simulink subsystem "PvtSubSys_VSM_LDW"  (R2020b)
settings: Solver=VariableStepAuto  StartTime=0.0  StopTime=10.0  RelTol=1e-3
values from neighbouring files (symbols this model uses):
  P_VSM_LDW_AbsEspInTime = 3.0    [LDW.sldd]
  P_VSM_LDW_absLongitudeAccIn = 2.5    [LDW.sldd]
  P_VSM_LDW_absLongitudeAccOut = 3.0    [LDW.sldd]
  P_VSM_LDW_AccPedalOut = 30.0    [LDW.sldd]
  P_VSM_LDW_AccRateIn = 30.0    [LDW.sldd]
  P_VSM_LDW_AccRateInTime = 1.5    [LDW.sldd]
  P_VSM_LDW_AccRateOut = 80.0    [LDW.sldd]
  P_VSM_LDW_AccRateOutTime = 0.0    [LDW.sldd]
  P_VSM_LDW_BrakePressIn = 3.0    [LDW.sldd]
  P_VSM_LDW_BrakePressInTime = 1.5    [LDW.sldd]
  P_VSM_LDW_BrakePressOut = 5.0    [LDW.sldd]
  P_VSM_LDW_LaneChangeOffset = 0.11    [LDW.sldd]
  P_VSM_LDW_LaneCurveIn = 0.005    [LDW.sldd]
  P_VSM_LDW_LaneCurveOut = 0.006    [LDW.sldd]
  P_VSM_LDW_LateralAcceIn = 3.0    [LDW.sldd]
  P_VSM_LDW_LateralAcceInTime = 3.0    [LDW.sldd]
  P_VSM_LDW_LateralAcceOut = 3.5    [LDW.sldd]
  P_VSM_LDW_LongitudeAccIn = 3.0    [LDW.sldd]
  P_VSM_LDW_LongitudeAccInTime = 3.0    [LDW.sldd]
  P_VSM_LDW_LongitudeAccOut = 3.5    [LDW.sldd]
  P_VSM_LDW_State_Absesp_enable = 1.0    [LDW.sldd]
  P_VSM_LDW_State_Accpedalrate_enable = 1.0    [LDW.sldd]
  P_VSM_LDW_State_Breakpressure_enable = 1.0    [LDW.sldd]
  P_VSM_LDW_State_ESSSts_enable = 1.0    [LDW.sldd]
  P_VSM_LDW_State_Failsafe_enable = 1.0    [LDW.sldd]
  P_VSM_LDW_State_GEAR_enable = 1.0    [LDW.sldd]
  P_VSM_LDW_State_Headingangle_enable = 1.0    [LDW.sldd]
  P_VSM_LDW_State_Lane_enable = 1.0    [LDW.sldd]
  P_VSM_LDW_State_LaneChange_enable = 1.0    [LDW.sldd]
  P_VSM_LDW_State_Lanecurve_enable = 1.0    [LDW.sldd]
  P_VSM_LDW_State_LateralAcce_enable = 1.0    [LDW.sldd]
  P_VSM_LDW_State_LongitudeAcc_enable = 1.0    [LDW.sldd]
  P_VSM_LDW_State_Param_LaneWidth_Offset : value not decoded    [LDW.sldd]
  P_VSM_LDW_State_Param_REWarningZoneIn = 0.35    [LDW.sldd]
  P_VSM_LDW_State_Param_Sensitive_Offset : value not decoded    [LDW.sldd]
  P_VSM_LDW_State_Param_WarningZoneIn = 0.2    [LDW.sldd]
  P_VSM_LDW_State_Param_WarningZoneOut = -0.65    [LDW.sldd]
  P_VSM_LDW_State_SteerWheelAngle_enable = 1.0    [LDW.sldd]
  P_VSM_LDW_State_SteerWheelSpd_enable = 1.0    [LDW.sldd]
  P_VSM_LDW_State_TurnLight_enable = 1.0    [LDW.sldd]
  P_VSM_LDW_State_Vehspeed_enable = 1.0    [LDW.sldd]
  P_VSM_LDW_State_Yawsup_enable = 1.0    [LDW.sldd]
  P_VSM_LDW_SteerWheelAngleIn = 70.0    [LDW.sldd]
  P_VSM_LDW_SteerWheelAngleInTime = 3.0    [LDW.sldd]
  P_VSM_LDW_SteerWheelAngleOut = 90.0    [LDW.sldd]
  P_VSM_LDW_SteerWheelSpdIn = 150.0    [LDW.sldd]
  P_VSM_LDW_SteerWheelSpdInTime = 3.0    [LDW.sldd]
  P_VSM_LDW_SteerWheelSpdOut = 200.0    [LDW.sldd]
  P_VSM_LDW_TurnLightInTime = 3.0    [LDW.sldd]
  P_VSM_LDW_WhelDy = 2.0    [LDW.sldd]
  P_VSM_LDW_YawRateIn = 0.2    [LDW.sldd]
  P_VSM_LDW_YawRateInTime = 1.0    [LDW.sldd]
  P_VSM_LDW_YawRateOut = 0.25    [LDW.sldd]
undefined symbols (not defined in the file or in its folder): P_VSM_LSMC_SampleTime
libraries: simulink x106
(part 2 of 3)

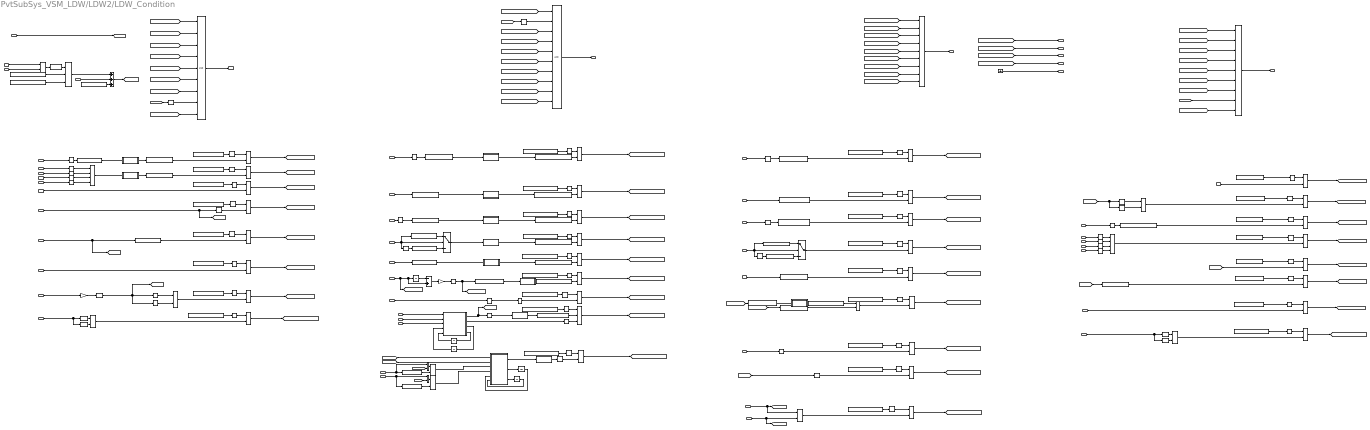
== system PvtSubSys_VSM_LDW/LDW2/LDW_Condition ==
  note: Ready2Active
  note: 0x0:Current gear "N" or "P"
      | 0x1:Current gear "1"
      | 0x2:Current gear "2"
      | 0x3:Current gear "3"
      | 0x4:Current gear "4"
      | 0x5:Current gear "5"
      | 0x6:Current gear "6"
      | 0x7:Current gear "7"
      | 0x8:Current gear "R"
      | 0x9-0xF:Reserved
  note: Active2Ready
  note: 0.2
  note: 0.35
  HWAActive : Inport
  canSASSteerWheelAngle : Inport  Port=2
  canSASSteerWheelSpd : Inport  Port=3
  canABMLateralAcce : Inport  Port=4
  LongitudeAcc : Inport  Port=5
  canESP_MasterCylindBrakePress : Inport  Port=6
  canECMAccrPedlPosnDiagc : Inport  Port=7
  CURRENT_GEAR : Inport  Port=8
  canBCMLeftTurnSWSts : Inport  Port=9
  canBCMRightTurnSWSts : Inport  Port=10
  Scene_LaneValid : Inport  Port=11
  canABMVehDynYawRate1 : Inport  Port=12
  canESPVDCActive1 : Inport  Port=13
  canESPPTCActive1 : Inport  Port=14
  canESPBTCActive1 : Inport  Port=15
  canABSABSActive1 : Inport  Port=16
  Common_Lane_Out : Inport  Port=17
  canABSVehicleSpd : Inport  Port=18
  Common_Lane_in : Inport  Port=19
  Headingangle_In : Inport  Port=20
  Headingangle_Out : Inport  Port=21
  LaneCurve : Inport  Port=22
  IFC_Failsafe : Inport  Port=23
  LeftChange : Inport  Port=24
  RightChange : Inport  Port=25
  FLWhelDy : Inport  Port=26
  FRWhelDy : Inport  Port=27
  ESSSts : Inport  Port=28
  LDWOffset : Inport  Port=29
  Host_LRE : Inport  Port=30
  Host_RRE : Inport  Port=31
  Abs{,1,3,6..8,11,15..16} (9 alike) : Abs
  Add : Sum  Inputs=-+
  Add1 : Sum  Inputs=+++
  Bias : Bias  Bias=1.3
  CURRENT_GEAR1 : InportShadow  Port=8
  Compare To Constant{1,19,24,28,32..33,38,42..44,46..48,56,69,78..79,82,88,115,118..119} (22 alike) : simulink/Logic and Bit Operations/Compare To Constant  relop===  const=1  OutDataTypeStr=boolean
  Compare To Constant{2,5..12,16..18,26..27,36,41,50..52,95,98,108,121,124} (24 alike) : simulink/Logic and Bit Operations/Compare To Constant  relop===  const=0  OutDataTypeStr=boolean
  Compare To Constant100 : simulink/Logic and Bit Operations/Compare To Constant  relop=<  const=P_VSM_LDW_LateralAcceIn  OutDataTypeStr=boolean
  Compare To Constant120 : simulink/Logic and Bit Operations/Compare To Constant  relop=>  const=P_VSM_LDW_AbsEspInTime  OutDataTypeStr=boolean
  Compare To Constant13 : simulink/Logic and Bit Operations/Compare To Constant  relop=>  const=0  OutDataTypeStr=boolean
  Compare To Constant14 : simulink/Logic and Bit Operations/Compare To Constant  relop=>  const=P_VSM_LDW_AccRateInTime  OutDataTypeStr=boolean
  Compare To Constant15 : simulink/Logic and Bit Operations/Compare To Constant  relop=>  const=P_VSM_LDW_TurnLightInTime  OutDataTypeStr=boolean
  Compare To Constant20 : simulink/Logic and Bit Operations/Compare To Constant  relop=<  const=P_VSM_LDW_BrakePressIn  OutDataTypeStr=boolean
  Compare To Constant21 : simulink/Logic and Bit Operations/Compare To Constant  relop===  const=8  OutDataTypeStr=boolean
  Compare To Constant22 : simulink/Logic and Bit Operations/Compare To Constant  relop=<  const=P_VSM_LDW_YawRateIn  OutDataTypeStr=boolean
  Compare To Constant23 : simulink/Logic and Bit Operations/Compare To Constant  relop=>  const=P_VSM_LDW_YawRateInTime  OutDataTypeStr=boolean
  Compare To Constant29 : simulink/Logic and Bit Operations/Compare To Constant  relop=<  const=P_VSM_LDW_SteerWheelAngleIn  OutDataTypeStr=boolean
  Compare To Constant3 : simulink/Logic and Bit Operations/Compare To Constant  relop=>  const=P_VSM_LDW_AccPedalOut  OutDataTypeStr=boolean
  Compare To Constant31 : simulink/Logic and Bit Operations/Compare To Constant  relop=<  const=P_VSM_LDW_SteerWheelSpdIn  OutDataTypeStr=boolean
  Compare To Constant35 : simulink/Logic and Bit Operations/Compare To Constant  relop=>  const=60  OutDataTypeStr=boolean
  Compare To Constant37 : simulink/Logic and Bit Operations/Compare To Constant  relop=<  const=150  OutDataTypeStr=boolean
  Compare To Constant39 : simulink/Logic and Bit Operations/Compare To Constant  relop=<  const=55  OutDataTypeStr=boolean
  Compare To Constant4 : simulink/Logic and Bit Operations/Compare To Constant  relop=>  const=P_VSM_LDW_AccRateOutTime  OutDataTypeStr=boolean
  Compare To Constant40 : simulink/Logic and Bit Operations/Compare To Constant  relop=>  const=155  OutDataTypeStr=boolean
  Compare To Constant49 : simulink/Logic and Bit Operations/Compare To Constant  relop=>  const=0.5  OutDataTypeStr=boolean
  Compare To Constant53 : simulink/Logic and Bit Operations/Compare To Constant  relop=~=  const=5  OutDataTypeStr=boolean
  Compare To Constant54 : simulink/Logic and Bit Operations/Compare To Constant  relop=<  const=P_VSM_LDW_WhelDy  OutDataTypeStr=boolean
  Compare To Constant55 : simulink/Logic and Bit Operations/Compare To Constant  relop=<  const=P_VSM_LDW_WhelDy  OutDataTypeStr=boolean
  Compare To Constant57 : simulink/Logic and Bit Operations/Compare To Constant  relop===  const=8  OutDataTypeStr=boolean
  Compare To Constant58 : simulink/Logic and Bit Operations/Compare To Constant  relop=<  const=P_VSM_LDW_LongitudeAccIn  OutDataTypeStr=boolean
  Compare To Constant59 : simulink/Logic and Bit Operations/Compare To Constant  relop=<  const=P_VSM_LDW_absLongitudeAccIn  OutDataTypeStr=boolean
  Compare To Constant60 : simulink/Logic and Bit Operations/Compare To Constant  relop===  const=5  OutDataTypeStr=boolean
  Compare To Constant61 : simulink/Logic and Bit Operations/Compare To Constant  relop=>  const=P_VSM_LDW_SteerWheelAngleOut  OutDataTypeStr=boolean
  Compare To Constant62 : simulink/Logic and Bit Operations/Compare To Constant  relop===  const=4  OutDataTypeStr=boolean
  Compare To Constant63 : simulink/Logic and Bit Operations/Compare To Constant  relop=<  const=P_VSM_LDW_LaneCurveIn  OutDataTypeStr=boolean
  Compare To Constant65 : simulink/Logic and Bit Operations/Compare To Constant  relop=>  const=P_VSM_LDW_SteerWheelAngleInTime  OutDataTypeStr=boolean
  Compare To Constant67 : simulink/Logic and Bit Operations/Compare To Constant  relop=~=  const=4  OutDataTypeStr=boolean
  Compare To Constant70 : simulink/Logic and Bit Operations/Compare To Constant  relop=>  const=P_VSM_LDW_YawRateOut  OutDataTypeStr=boolean
  Compare To Constant73 : simulink/Logic and Bit Operations/Compare To Constant  relop=>  const=P_VSM_LDW_SteerWheelSpdOut  OutDataTypeStr=boolean
  Compare To Constant74 : simulink/Logic and Bit Operations/Compare To Constant  relop=>  const=P_VSM_LDW_SteerWheelSpdInTime  OutDataTypeStr=boolean
  Compare To Constant75 : simulink/Logic and Bit Operations/Compare To Constant  relop=>  const=P_VSM_LDW_LateralAcceOut  OutDataTypeStr=boolean
  Compare To Constant76 : simulink/Logic and Bit Operations/Compare To Constant  relop=>  const=P_VSM_LDW_LongitudeAccOut  OutDataTypeStr=boolean
  Compare To Constant77 : simulink/Logic and Bit Operations/Compare To Constant  relop=>  const=P_VSM_LDW_absLongitudeAccOut  OutDataTypeStr=boolean
  Compare To Constant80 : simulink/Logic and Bit Operations/Compare To Constant  relop=>  const=P_VSM_LDW_BrakePressOut  OutDataTypeStr=boolean
  Compare To Constant83 : simulink/Logic and Bit Operations/Compare To Constant  relop=>  const=P_VSM_LDW_AccRateOut  OutDataTypeStr=boolean
  Compare To Constant85 : simulink/Logic and Bit Operations/Compare To Constant  relop=>  const=P_VSM_LDW_LaneCurveOut  OutDataTypeStr=boolean
  Compare To Constant91 : simulink/Logic and Bit Operations/Compare To Constant  relop=<  const=P_VSM_LDW_AccRateIn  OutDataTypeStr=boolean
  Compare To Constant92 : simulink/Logic and Bit Operations/Compare To Constant  relop=>  const=P_VSM_LDW_BrakePressInTime  OutDataTypeStr=boolean
  Compare To Constant94 : simulink/Logic and Bit Operations/Compare To Constant  relop=>  const=P_VSM_LDW_LongitudeAccInTime  OutDataTypeStr=boolean
  Compare To Constant96 : simulink/Logic and Bit Operations/Compare To Constant  relop=>  const=P_VSM_LDW_LateralAcceInTime  OutDataTypeStr=boolean
  Constant : Constant  Value=P_VSM_LDW_LaneChangeOffset
  Data Type Conversion : DataTypeConversion
  ESSSts2 : InportShadow  Port=28
  Gain : Gain  Gain=1.03
  Gain1 : Gain  Gain=50
  Ground : Ground
  Logical Operator{,3,5,7,9..12,15,17,19..20,24..26,38..41,46,60,62} (22 alike) : Logic  AllPortsSameDT=off  OutDataTypeStr=boolean
  Logical Operator1 : Logic  Inputs=4  AllPortsSameDT=off  OutDataTypeStr=boolean
  Logical Operator13 : Logic  Operator=OR  Inputs=4  AllPortsSameDT=off  OutDataTypeStr=boolean
  Logical Operator{4,6,8,16,18,21..22,27,29..32,34,36..37,42,49,52,59,61} (20 alike) : Logic  Operator=OR  AllPortsSameDT=off  OutDataTypeStr=boolean
  Logical Operator23 : Logic  Operator=NOT  AllPortsSameDT=off  OutDataTypeStr=boolean
  Logical Operator35 : Logic  Operator=NOT  AllPortsSameDT=off  OutDataTypeStr=boolean
  Logical Operator43 : Logic  Operator=OR  Inputs=9  AllPortsSameDT=off  OutDataTypeStr=boolean
  Logical Operator45 : Logic  Operator=OR  Inputs=9  AllPortsSameDT=off  OutDataTypeStr=boolean
  Logical Operator51 : Logic  Operator=OR  Inputs=3  AllPortsSameDT=off  OutDataTypeStr=boolean
  Logical Operator86 : Logic  Inputs=9  AllPortsSameDT=off  OutDataTypeStr=boolean
  Logical Operator94 : Logic  Inputs=10  AllPortsSameDT=off  OutDataTypeStr=boolean
  LongitudeAcc1 : InportShadow  Port=5
  MATLAB Function : MATLAB Function  TreatAsAtomicUnit=on
  Multiport Switch : MultiPortSwitch  Inputs=2  DiagnosticForDefault=None
  Relational Operator : RelationalOperator  OutDataTypeStr=boolean  RndMeth=Simplest
  Relational Operator1 : RelationalOperator  OutDataTypeStr=boolean  RndMeth=Simplest
  State_TurnLight2 : MATLAB Function  TreatAsAtomicUnit=on
  Subsystem : Subsystem  mask{Ts=P_VSM_LSMC_SampleTime, Max=10}
      mask prompts: Ts "Sample Time:"; Max "Max Limit:"
      mask Display:
      | Ts=get_param(gcb,'Ts');
      | Max=get_param(gcb,'Max');
      | disp(['Ts:' Ts '\n' 'Max:' Max ]);
  Subsystem1 : Subsystem  mask{Ts=P_VSM_LSMC_SampleTime, Max=10}
      mask prompts: Ts "Sample Time:"; Max "Max Limit:"
      mask Display:
      | Ts=get_param(gcb,'Ts');
      | Max=get_param(gcb,'Max');
      | disp(['Ts:' Ts '\n' 'Max:' Max ]);
  Subsystem10 : Subsystem  mask{Ts=P_VSM_LSMC_SampleTime, Max=10}
      mask prompts: Ts "Sample Time:"; Max "Max Limit:"
      mask Display:
      | Ts=get_param(gcb,'Ts');
      | Max=get_param(gcb,'Max');
      | disp(['Ts:' Ts '\n' 'Max:' Max ]);
  Subsystem17 : Subsystem  mask{Ts=P_VSM_LSMC_SampleTime, Max=10}
      mask prompts: Ts "Sample Time:"; Max "Max Limit:"
      mask Display:
      | Ts=get_param(gcb,'Ts');
      | Max=get_param(gcb,'Max');
      | disp(['Ts:' Ts '\n' 'Max:' Max ]);
  Subsystem2 : Subsystem  mask{Ts=P_VSM_LSMC_SampleTime, Max=10}
      mask prompts: Ts "Sample Time:"; Max "Max Limit:"
      mask Display:
      | Ts=get_param(gcb,'Ts');
      | Max=get_param(gcb,'Max');
      | disp(['Ts:' Ts '\n' 'Max:' Max ]);
  Subsystem3 : Subsystem  mask{Ts=P_VSM_LSMC_SampleTime, Max=10}
      mask prompts: Ts "Sample Time:"; Max "Max Limit:"
      mask Display:
      | Ts=get_param(gcb,'Ts');
      | Max=get_param(gcb,'Max');
      | disp(['Ts:' Ts '\n' 'Max:' Max ]);
  Subsystem4 : Subsystem  mask{Ts=P_VSM_LSMC_SampleTime, Max=10}
      mask prompts: Ts "Sample Time:"; Max "Max Limit:"
      mask Display:
      | Ts=get_param(gcb,'Ts');
      | Max=get_param(gcb,'Max');
      | disp(['Ts:' Ts '\n' 'Max:' Max ]);
  Subsystem5 : Subsystem  mask{Ts=P_VSM_LSMC_SampleTime, Max=10}
      mask prompts: Ts "Sample Time:"; Max "Max Limit:"
      mask Display:
      | Ts=get_param(gcb,'Ts');
      | Max=get_param(gcb,'Max');
      | disp(['Ts:' Ts '\n' 'Max:' Max ]);
  Subsystem6 : Subsystem  mask{Ts=P_VSM_LSMC_SampleTime, Max=10}
      mask prompts: Ts "Sample Time:"; Max "Max Limit:"
      mask Display:
      | Ts=get_param(gcb,'Ts');
      | Max=get_param(gcb,'Max');
      | disp(['Ts:' Ts '\n' 'Max:' Max ]);
  Subsystem7 : Subsystem  mask{Ts=P_VSM_LSMC_SampleTime, Max=10}
      mask prompts: Ts "Sample Time:"; Max "Max Limit:"
      mask Display:
      | Ts=get_param(gcb,'Ts');
      | Max=get_param(gcb,'Max');
      | disp(['Ts:' Ts '\n' 'Max:' Max ]);
  Subsystem8 : Subsystem  mask{Ts=P_VSM_LSMC_SampleTime, Max=10}
      mask prompts: Ts "Sample Time:"; Max "Max Limit:"
      mask Display:
      | Ts=get_param(gcb,'Ts');
      | Max=get_param(gcb,'Max');
      | disp(['Ts:' Ts '\n' 'Max:' Max ]);
  Switch2 : Switch  Criteria=u2 > Threshold
  Switch4 : Switch  Criteria=u2 > Threshold
  Unit Delay{1..4,8} (5 alike) : UnitDelay  SampleTime=-1  HasFrameUpgradeWarning=on
  WarningZoneIn : Constant  Value=P_VSM_LDW_State_Param_WarningZoneIn
  WarningZoneIn1 : Constant  Value=P_VSM_LDW_State_Param_REWarningZoneIn
  canABMLateralAcce2 : InportShadow  Port=4
  canABMVehDynYawRate2 : InportShadow  Port=12
  canABSABSActive2 : InportShadow  Port=16
  canESPBTCActive2 : InportShadow  Port=15
  canESPPTCActive2 : InportShadow  Port=14
  canESPVDCActive2 : InportShadow  Port=13
  canESP_MasterCylindBrakePress2 : InportShadow  Port=6
  canSASSteerWheelAngle1 : InportShadow  Port=2
  canSASSteerWheelSpd2 : InportShadow  Port=3
  param_1 : Constant  Value=P_VSM_LDW_State_SteerWheelAngle_enable
  param_10 : Constant  Value=P_VSM_LDW_State_Headingangle_enable
  param_11 : Constant  Value=P_VSM_LDW_State_Breakpressure_enable
  param_13 : Constant  Value=P_VSM_LDW_State_Accpedalrate_enable
  param_14 : Constant  Value=P_VSM_LDW_State_Absesp_enable
  param_15 : Constant  Value=P_VSM_LDW_State_Failsafe_enable
  param_17 : Constant  Value=P_VSM_LDW_State_Lanecurve_enable
  param_18 : Constant  Value=P_VSM_LDW_State_GEAR_enable
  param_19 : Constant  Value=P_VSM_LDW_State_ESSSts_enable
  param_2 : Constant  Value=P_VSM_LDW_State_LaneChange_enable
  param_20 : Constant  Value=P_VSM_LDW_State_TurnLight_enable
  param_23 : Constant  Value=P_VSM_LDW_State_SteerWheelSpd_enable
  param_24 : Constant  Value=P_VSM_LDW_State_LateralAcce_enable
  param_25 : Constant  Value=P_VSM_LDW_State_Vehspeed_enable
  param_26 : Constant  Value=P_VSM_LDW_State_Yawsup_enable
  param_27 : Constant  Value=P_VSM_LDW_State_Absesp_enable
  param_28 : Constant  Value=P_VSM_LDW_State_LongitudeAcc_enable
  param_29 : Constant  Value=P_VSM_LDW_State_Lane_enable
  param_3 : Constant  Value=P_VSM_LDW_State_Yawsup_enable
  param_30 : Constant  Value=P_VSM_LDW_State_Failsafe_enable
  param_31 : Constant  Value=P_VSM_LDW_State_Breakpressure_enable
  param_32 : Constant  Value=P_VSM_LDW_State_Headingangle_enable
  param_33 : Constant  Value=P_VSM_LDW_State_Lanecurve_enable
  param_4 : Constant  Value=P_VSM_LDW_State_SteerWheelAngle_enable
  param_40 : Constant  Value=P_VSM_LDW_State_Lane_enable
  param_42 : Constant  Value=P_VSM_LDW_State_Vehspeed_enable
  param_43 : Constant  Value=P_VSM_LDW_State_Accpedalrate_enable
  param_45 : Constant  Value=P_VSM_LDW_State_GEAR_enable
  param_46 : Constant  Value=P_VSM_LDW_State_TurnLight_enable
  param_47 : Constant  Value=P_VSM_LDW_State_LaneChange_enable
  param_6 : Constant  Value=P_VSM_LDW_State_SteerWheelSpd_enable
  param_7 : Constant  Value=P_VSM_LDW_State_LateralAcce_enable
  param_8 : Constant  Value=P_VSM_LDW_State_ESSSts_enable
  param_9 : Constant  Value=P_VSM_LDW_State_LongitudeAcc_enable
  LDW_Idle2Ready : Outport
  LDW_Ready2Active : Outport  Port=2
  LDW_Active2Ready : Outport  Port=3
  LDW_Ready2Idle_Active2Idle : Outport  Port=4
  LDW_Con_AccPedalRate_LDWExit : Outport  Port=5
  LDW_Con_BrakePressure_ LDWExit : Outport  Port=6
  LDW_Con_SteerWheelSpd_ LDWExit : Outport  Port=7
  LDW_Con_SteerWheelAngle_ LDWExit : Outport  Port=8
  LDW_Con_DriverInput_ LDWExit : Outport  Port=9
  wires:
  LDWOffset/1 -> Add1/2
  [Con_AccPedalRate_Active2Ready] -> LDW_Con_AccPedalRate_LDWExit/1  "LDW_Con_AccPedalRate_LDWExit"
  Ground/1 -> LDW_Con_DriverInput_ LDWExit/1  "LDW_Con_DriverInput_ LDWExit"
  [Con_SteerWheelAngle_Active2Ready] -> LDW_Con_SteerWheelAngle_ LDWExit/1  "LDW_Con_SteerWheelAngle_ LDWExit"
  [Con_SteerWheelSpd_Active2Ready] -> LDW_Con_SteerWheelSpd_ LDWExit/1  "LDW_Con_SteerWheelSpd_ LDWExit"
  [Con_BrakePressure_Active2Ready] -> LDW_Con_BrakePressure_ LDWExit/1  "LDW_Con_BrakePressure_ LDWExit"
  [Con_SteerWheelSpd_Ready2Active] -> Logical Operator94/3
  [Con_BrakePressure_Ready2Active] -> Logical Operator94/6
  [Con_LateralAcc_Ready2Active] -> Logical Operator94/4
  [Con_AccPedalRate_Ready2Active] -> Logical Operator94/7
  [Con_SteerWheelAngle_Ready2Active] -> Logical Operator94/1
  canBCMLeftTurnSWSts/1 -> State_TurnLight2/1(leftlight)
  Compare To Constant42/1 -> Logical Operator10/1
  Compare To Constant2/1 -> Logical Operator27/1
  Compare To Constant13/1 -> Logical Operator15/2
  Compare To Constant47/1 -> Logical Operator15/1
  Logical Operator27/1 -> [Con_SteerWheelAngle_Ready2Active]  "VSM_LDW_Con_SteerWheelAngle_Ready2Active"
  Logical Operator17/1 -> [Con_CURRENT_GEAR_Active2Ready]  "VSM_LDW_Con_CURRENT_GEAR_Active2Ready"
  Compare To Constant27/1 -> Logical Operator51/1
  LongitudeAcc/1 -> Switch2/2, Compare To Constant58/1, Abs7/1
  Compare To Constant59/1 -> Switch2/3
  Logical Operator3/1 -> [Con_SteerWheelSpd_Active2Ready]  "VSM_LDW_Con_SteerWheelSpd_Active2Ready"
  Compare To Constant8/1 -> Logical Operator31/1
  canSASSteerWheelAngle1/1 -> Abs8/1
  Abs16/1 -> Compare To Constant75/1
  CURRENT_GEAR1/1 -> Compare To Constant57/1
  Logical Operator11/1 -> [Con_BrakePressure_Active2Ready]  "VSM_LDW_Con_BrakePressure_Active2Ready"
  param_20/1 -> Compare To Constant27/1
  Switch4/1 -> Logical Operator10/2
  Logical Operator35/1 -> Logical Operator37/2
  Compare To Constant77/1 -> Switch4/3
  LongitudeAcc1/1 -> Abs15/1, Compare To Constant76/1, Switch4/2
  Abs3/1 -> [AccrPedlPosnRate], Compare To Constant91/1
  Compare To Constant124/1 -> Logical Operator52/1
  Logical Operator31/1 -> [Con_SteerWheelSpd_Ready2Active]  "VSM_LDW_Con_SteerWheelSpd_Ready2Active"
  Abs7/1 -> Compare To Constant59/1
  Abs8/1 -> Compare To Constant61/1
  canESP_MasterCylindBrakePress2/1 -> Compare To Constant80/1
  [AccrPedlPosnRate] -> Compare To Constant83/1
  Compare To Constant33/1 -> Logical Operator12/1
  Compare To Constant78/1 -> Logical Operator11/1
  CURRENT_GEAR/1 -> Compare To Constant21/1
  Compare To Constant75/1 -> Logical Operator7/2
  Logical Operator10/1 -> [Con_LongitudeAcc_Active2Ready]  "VSM_LDW_Con_LongitudeAcc_Active2Ready"
  Compare To Constant46/1 -> Logical Operator38/1
  Logical Operator37/1 -> [Con_CURRENT_GEAR_Ready2Active]  "VSM_LDW_Con_CURRENT_GEAR_Ready2Active"
  Abs1/1 -> Compare To Constant29/1
  Compare To Constant58/1 -> Switch2/1
  param_1/1 -> Compare To Constant2/1
  Logical Operator7/1 -> [Con_LateralAcc_Active2Ready]  "VSM_LDW_Con_LateralAcc_Active2Ready"
  Compare To Constant61/1 -> Logical Operator38/2
  Compare To Constant21/1 -> Logical Operator35/1
  canBCMRightTurnSWSts/1 -> State_TurnLight2/2(rightlight)
  canESP_MasterCylindBrakePress/1 -> Compare To Constant20/1
  canABMLateralAcce2/1 -> Abs16/1
  Abs11/1 -> Compare To Constant100/1
  Logical Operator49/1 -> [Con_BrakePressure_Ready2Active]  "VSM_LDW_Con_BrakePressure_Ready2Active"
  Compare To Constant121/1 -> Logical Operator49/1
  Abs15/1 -> Compare To Constant77/1
  canSASSteerWheelSpd2/1 -> Compare To Constant73/1
  canABMLateralAcce/1 -> Abs11/1
  Compare To Constant11/1 -> Logical Operator34/1
  Logical Operator52/1 -> [Con_AccPedalRate_Ready2Active]  "VSM_LDW_Con_AccPedalRate_Ready2Active"
  param_6/1 -> Compare To Constant8/1
  Logical Operator38/1 -> [Con_SteerWheelAngle_Active2Ready]  "VSM_LDW_Con_SteerWheelAngle_Active2Ready"
  [Con_LongitudeAcc_Ready2Active] -> Logical Operator94/5
  Compare To Constant73/1 -> Logical Operator3/2
  Logical Operator32/1 -> [Con_LateralAcc_Ready2Active]  "VSM_LDW_Con_LateralAcc_Ready2Active"
  Compare To Constant48/1 -> Logical Operator17/1
  Logical Operator34/1 -> [Con_LongitudeAcc_Ready2Active]  "VSM_LDW_Con_LongitudeAcc_Ready2Active"
  Logical Operator51/1 -> [Con_TurnLight_Ready2Active]  "VSM_LDW_Con_TurnLight_Ready2Active"
  Compare To Constant43/1 -> Logical Operator7/1
  canSASSteerWheelSpd/1 -> Compare To Constant31/1
  Compare To Constant26/1 -> Logical Operator37/1
  Compare To Constant9/1 -> Logical Operator32/1
  [Turnlight] -> Compare To Constant13/1
  Logical Operator15/1 -> [Con_TurnLight_Active2Ready]  "VSM_LDW_Con_TurnLight_Active2Ready"
  [Con_LateralAcc_Active2Ready] -> Logical Operator45/4
  Compare To Constant76/1 -> Switch4/1
  [Con_LaneChange_Active2Ready] -> Logical Operator45/8
  [Con_AccPedalRate_Active2Ready] -> Logical Operator45/7
  Logical Operator12/1 -> [Con_AccPedalRate_Active2Ready]  "VSM_LDW_Con_AccPedalRate_Active2Ready"
  [Con_BrakePressure_Active2Ready] -> Logical Operator45/6
  [Con_CURRENT_GEAR_Active2Ready] -> Logical Operator45/2
  [Con_SteerWheelSpd_Active2Ready] -> Logical Operator45/3
  canSASSteerWheelAngle/1 -> Abs1/1
  [Con_SteerWheelAngle_Active2Ready] -> Logical Operator45/1
  Compare To Constant44/1 -> Logical Operator3/1
  [Con_LongitudeAcc_Active2Ready] -> Logical Operator45/5
  Compare To Constant57/1 -> Logical Operator17/2
  param_4/1 -> Compare To Constant46/1
  param_17/1 -> Compare To Constant115/1
  Logical Operator46/1 -> [Con_LaneCurve_Ready2Idle]  "VSM_LDW_Con_LaneCurve_Ready2Idle"
  Compare To Constant85/1 -> Logical Operator46/2
  Headingangle_Out/1 -> Logical Operator26/2
  Logical Operator26/1 -> [Con_Headingangle_Ready2Idle]  "VSM_LDW_Con_Headingangle_Ready2Idle"
  param_32/1 -> Compare To Constant32/1
  Compare To Constant40/1 -> Logical Operator61/2
  param_25/1 -> Compare To Constant38/1
  canABSABSActive1/1 -> Compare To Constant69/1
  canESPVDCActive1/1 -> Compare To Constant79/1
  Compare To Constant19/1 -> Logical Operator9/1
  Logical Operator39/1 -> [Con_YawRate_Ready2Idle]  "VSM_LDW_Con_YawRate_Ready2Idle"
  Logical Operator24/1 -> [Con_Failsafe_Ready2Idle]  "VSM_LDW_Con_Failsafe_Ready2Idle"
  Logical Operator40/1 -> [Con_AbsEsp_Ready2Idle]  "VSM_LDW_Con_AbsEsp_Ready2Idle"
  Compare To Constant39/1 -> Logical Operator61/1
  param_29/1 -> Compare To Constant19/1
  Compare To Constant115/1 -> Logical Operator46/1
  Compare To Constant88/1 -> Logical Operator13/3
  Compare To Constant70/1 -> Logical Operator39/2
  [IFC_Failsafe] -> Logical Operator24/2
  canABMVehDynYawRate1/1 -> Abs6/1
  Abs6/1 -> Compare To Constant70/1
  Logical Operator62/1 -> [Con_VehicleSpeed_Ready2Idle]  "VSM_LDW_Con_VehicleSpeed_Ready2Idle"
  Compare To Constant32/1 -> Logical Operator26/1
  Compare To Constant69/1 -> Logical Operator13/4
  param_30/1 -> Compare To Constant28/1
  canESPBTCActive1/1 -> Compare To Constant88/1
  Compare To Constant119/1 -> Logical Operator40/1
  param_27/1 -> Compare To Constant119/1
  Logical Operator13/1 -> Logical Operator40/2  "absespsup"
  Compare To Constant38/1 -> Logical Operator62/1
  Compare To Constant118/1 -> Logical Operator39/1
  Common_Lane_Out/1 -> Logical Operator9/2
  Logical Operator9/1 -> [Con_Lane_Ready2Idle]  "VSM_LDW_Con_Lane_Ready2Idle"
  param_26/1 -> Compare To Constant118/1
  Compare To Constant79/1 -> Logical Operator13/1
  Logical Operator61/1 -> Logical Operator62/2
  [LaneCurve] -> Compare To Constant85/1
  [Con_AbsEsp_Ready2Idle] -> Logical Operator43/2
  [speed] -> Compare To Constant39/1, Compare To Constant40/1
  [Con_Failsafe_Ready2Idle] -> Logical Operator43/3
  Compare To Constant82/1 -> Logical Operator13/2
  Compare To Constant28/1 -> Logical Operator24/1
  [Con_Headingangle_Ready2Idle] -> Logical Operator43/5
  [Con_YawRate_Ready2Idle] -> Logical Operator43/1
  canESPPTCActive1/1 -> Compare To Constant82/1
  Logical Operator43/1 -> LDW_Ready2Idle_Active2Idle/1  "VSM_LDW_Other2Idle"
  [Con_LaneCurve_Ready2Idle] -> Logical Operator43/4
  canABSVehicleSpd/1 -> Gain/1
  Logical Operator23/1 -> Logical Operator8/2
  [Con_Headingangel_Idle2Ready] -> Logical Operator86/3
  Common_Lane_in/1 -> Logical Operator4/2
  [Con_Failsafe_Idle2Ready] -> Logical Operator86/4
  Logical Operator86/1 -> LDW_Idle2Ready/1  "VSM_LDW_Idle2Ready"
  Compare To Constant35/1 -> Logical Operator60/1
  [Con_AbsEsp_Idle2Ready] -> Logical Operator86/2
  [Con_YawRate_Idle2Ready] -> Logical Operator86/1
  param_40/1 -> Compare To Constant16/1
  Logical Operator6/1 -> [Con_Headingangel_Idle2Ready]  "VSM_LDW_Con_Headingangle_Idle2Ready"
  Compare To Constant18/1 -> Logical Operator8/1
  param_15/1 -> Compare To Constant18/1
  Subsystem17/1(Out1) -> Compare To Constant120/1
  canABMVehDynYawRate2/1 -> Abs/1
  canESPBTCActive2/1 -> Compare To Constant7/1
  Subsystem/1(Out1) -> Compare To Constant23/1
  Compare To Constant22/1 -> Subsystem/1(In1)
  IFC_Failsafe/1 -> [IFC_Failsafe], Logical Operator23/1
  Logical Operator59/1 -> [Con_VehicleSpeed_Idle2Ready]  "VSM_LDW_Con_VehicleSpeed_Idle2Ready"
  param_33/1 -> Compare To Constant108/1
  Logical Operator29/1 -> [Con_YawRate_Idle2Ready]  "VSM_LDW_Con_YawRate_Idle2Ready"
  Logical Operator8/1 -> [Con_Failsafe_Idle2Ready]  "VSM_LDW_Con_Failsafe_Idle2Ready"
  Compare To Constant16/1 -> Logical Operator4/1
  Compare To Constant17/1 -> Logical Operator6/1
  canABSABSActive2/1 -> Compare To Constant10/1
  Compare To Constant5/1 -> Logical Operator1/1
  param_10/1 -> Compare To Constant17/1
  Compare To Constant6/1 -> Logical Operator1/2
  Compare To Constant7/1 -> Logical Operator1/3
  canESPVDCActive2/1 -> Compare To Constant5/1
  param_42/1 -> Compare To Constant36/1
  Logical Operator1/1 -> Subsystem17/1(In1)
  Compare To Constant95/1 -> Logical Operator29/1
  Bias/1 -> Compare To Constant35/1, Compare To Constant37/1, [speed]
  Compare To Constant37/1 -> Logical Operator60/2
  Compare To Constant36/1 -> Logical Operator59/1
  canESPPTCActive2/1 -> Compare To Constant6/1
  Logical Operator4/1 -> [Con_Lane_Idle2Ready]  "VSM_LDW_Con_Lane_Idle2Ready"
  Abs/1 -> Compare To Constant22/1
  param_3/1 -> Compare To Constant95/1
  Logical Operator36/1 -> [Con_LaneCurve_Idle2Ready]  "VSM_LDW_Con_LaneCurve_Idle2Ready"
  Compare To Constant108/1 -> Logical Operator36/1
  Compare To Constant98/1 -> Logical Operator30/1
  Logical Operator30/1 -> [Con_AbsEsp_Idle2Ready]  "VSM_LDW_Con_AbsEsp_Idle2Ready"
  LaneCurve/1 -> Compare To Constant63/1, [LaneCurve]
  Compare To Constant23/1 -> Logical Operator29/2
  Compare To Constant120/1 -> Logical Operator30/2
  Logical Operator60/1 -> Logical Operator59/2  "LogicalOperator60"
  Gain/1 -> Bias/1
  param_14/1 -> Compare To Constant98/1
  Compare To Constant63/1 -> Logical Operator36/2
  Compare To Constant10/1 -> Logical Operator1/4
  Logical Operator45/1 -> LDW_Active2Ready/1  "VSM_LDW_Active2Ready"
  Logical Operator94/1 -> LDW_Ready2Active/1  "VSM_LDW_Ready2Active"
  [Con_VehicleSpeed_Ready2Idle] -> Logical Operator43/6
  [Con_Lane_Ready2Idle] -> Logical Operator43/7
  Headingangle_In/1 -> Logical Operator6/2
  Compare To Constant15/1 -> Logical Operator51/2
  Compare To Constant12/1 -> Subsystem1/1(In1)
  Subsystem1/1(Out1) -> Compare To Constant15/1
  Compare To Constant14/1 -> Logical Operator52/2
  Compare To Constant80/1 -> Logical Operator11/2
  Compare To Constant92/1 -> Logical Operator49/2
  Compare To Constant94/1 -> Logical Operator34/2
  Compare To Constant91/1 -> Subsystem3/1(In1)
  Subsystem3/1(Out1) -> Compare To Constant14/1
  Compare To Constant20/1 -> Subsystem4/1(In1)
  Subsystem4/1(Out1) -> Compare To Constant92/1
  Switch2/1 -> Subsystem6/1(In1)
  Subsystem6/1(Out1) -> Compare To Constant94/1
  Compare To Constant96/1 -> Logical Operator32/2
  Compare To Constant100/1 -> Subsystem7/1(In1)
  Subsystem7/1(Out1) -> Compare To Constant96/1
  Compare To Constant74/1 -> Logical Operator31/2
  Subsystem10/1(Out1) -> Compare To Constant74/1
  Compare To Constant31/1 -> Subsystem10/1(In1)
  Compare To Constant65/1 -> Logical Operator27/2
  Compare To Constant29/1 -> Subsystem8/1(In1)
  Subsystem8/1(Out1) -> Compare To Constant65/1
  Compare To Constant24/1 -> Logical Operator5/1
  Logical Operator5/1 -> [Con_LaneChange_Active2Ready]  "VSM_LDW_Con_LaneChange_Active2Ready"
  Compare To Constant41/1 -> Logical Operator18/1
  Logical Operator18/1 -> [Con_LaneChange_Ready2Active]  "VSM_LDW_Con_LaneChange_Ready2Active"
  [Con_LaneCurve_Idle2Ready] -> Logical Operator86/5
  [Con_Lane_Idle2Ready] -> Logical Operator86/6
  [Con_VehicleSpeed_Idle2Ready] -> Logical Operator86/7
  Add/1 -> Gain1/1
  Gain1/1 -> Abs3/1
  Unit Delay4/1 -> Add/1
  [Con_CURRENT_GEAR_Ready2Active] -> Logical Operator94/8
  [Con_TurnLight_Ready2Active] -> Logical Operator94/9
  Compare To Constant1/1 -> Logical Operator51/3
  [Con_LaneChange_Ready2Active] -> Logical Operator94/10
  State_TurnLight2/3(left) -> Unit Delay8/1
  Unit Delay8/1 -> State_TurnLight2/4(leftk1)
  State_TurnLight2/4(right) -> Unit Delay1/1
  Unit Delay1/1 -> State_TurnLight2/5(rightk1)
  Scene_LaneValid/1 -> State_TurnLight2/3(lane)
  param_7/1 -> Compare To Constant9/1
  param_9/1 -> Compare To Constant11/1
  param_11/1 -> Compare To Constant121/1
  param_13/1 -> Compare To Constant124/1
  param_18/1 -> Compare To Constant26/1
  param_2/1 -> Compare To Constant41/1
  param_23/1 -> Compare To Constant44/1
  param_24/1 -> Compare To Constant43/1
  param_28/1 -> Compare To Constant42/1
  param_31/1 -> Compare To Constant78/1
  param_43/1 -> Compare To Constant33/1
  param_45/1 -> Compare To Constant48/1
  param_46/1 -> Compare To Constant47/1
  param_47/1 -> Compare To Constant24/1
  State_TurnLight2/1(state) -> [Turnlight], Compare To Constant12/1
  State_TurnLight2/2(out) -> Compare To Constant1/1
  HWAActive/1 -> [HWAActive]
  [HWAActive] -> Compare To Constant50/1
  Compare To Constant50/1 -> Logical Operator86/8
  Compare To Constant51/1 -> Logical Operator94/2
  [HWAActive] -> Compare To Constant51/1
  [HWAActive] -> Logical Operator43/8
  FLWhelDy/1 -> Compare To Constant55/1, Relational Operator/1
  FRWhelDy/1 -> Relational Operator1/1, Compare To Constant54/1
  MATLAB Function/1(y) -> Subsystem2/1(In1)  "LaneChangeR2A"
  [LeftChange] -> MATLAB Function/1(LeftChangefg)
  [RightChange] -> MATLAB Function/2(RightChangefg)
  Unit Delay3/1 -> MATLAB Function/6(Rfgk1)
  MATLAB Function/2(Lfg) -> Unit Delay2/1
  MATLAB Function/3(Rfg) -> Unit Delay3/1
  Unit Delay2/1 -> MATLAB Function/5(Lfgk1)
  LeftChange/1 -> [LeftChange], Logical Operator16/1
  RightChange/1 -> Logical Operator16/2, [RightChange]
  Logical Operator16/1 -> Logical Operator5/2
  Subsystem2/1(Out1) -> Compare To Constant49/1
  Compare To Constant49/1 -> Logical Operator18/2
  Compare To Constant54/1 -> Logical Operator19/2
  Relational Operator1/1 -> Logical Operator19/1
  Logical Operator19/1 -> MATLAB Function/4(Rdy)  "LDW_Rdy"
  Relational Operator/1 -> Logical Operator20/1
  Compare To Constant55/1 -> Logical Operator20/2
  Logical Operator20/1 -> MATLAB Function/3(Ldy)  "LDW_Ldy"
  Multiport Switch/1 -> Add1/1
  Add1/1 -> [ReactionIn]
  Host_RRE/1 -> Logical Operator21/2
  Logical Operator21/1 -> Data Type Conversion/1
  Data Type Conversion/1 -> Multiport Switch/1
  WarningZoneIn/1 -> Multiport Switch/3
  Host_LRE/1 -> Logical Operator21/1
  WarningZoneIn1/1 -> Multiport Switch/2
  [ReactionIn] -> Relational Operator/2
  [ReactionIn] -> Relational Operator1/2
  Constant/1 -> Add1/3
  Logical Operator22/1 -> [Con_ESSSts_Idle2Ready]  "VSM_LDW_Con_ESSSts_Idle2Ready"
  Compare To Constant67/1 -> Logical Operator25/1
  Logical Operator25/1 -> Logical Operator22/2
  Compare To Constant52/1 -> Logical Operator22/1
  param_8/1 -> Compare To Constant52/1
  Compare To Constant53/1 -> Logical Operator25/2
  ESSSts/1 -> Compare To Constant53/1, Compare To Constant67/1
  ESSSts2/1 -> Compare To Constant62/1, Compare To Constant60/1
  Compare To Constant60/1 -> Logical Operator42/2
  param_19/1 -> Compare To Constant56/1
  Compare To Constant56/1 -> Logical Operator41/1
  Logical Operator42/1 -> Logical Operator41/2
  Compare To Constant62/1 -> Logical Operator42/1
  Logical Operator41/1 -> [Con_ESSSts_Ready2Idle]  "VSM_LDW_Con_ESSSts_Ready2Idle"
  [Con_ESSSts_Ready2Idle] -> Logical Operator43/9
  [Con_ESSSts_Idle2Ready] -> Logical Operator86/9
  [Con_TurnLight_Active2Ready] -> Logical Operator45/9
  canECMAccrPedlPosnDiagc/1 -> [AccrPedlPosn], Unit Delay4/1, Add/2
  [AccrPedlPosn] -> Compare To Constant3/1
  Logical Operator/1 -> Logical Operator12/2
  Compare To Constant3/1 -> Logical Operator/2
  Subsystem5/1(Out1) -> Compare To Constant4/1
  Compare To Constant83/1 -> Subsystem5/1(In1)
  Compare To Constant4/1 -> Logical Operator/1
